simulink library "did"  (R2021b)
settings: Solver=VariableStepAuto  StartTime=0.0  StopTime=10.0  RelTol=1e-3
undefined symbols (not defined in the file): ADID_DODRange_pct, ADID_SOCRange_pct, ADID_TempRange_C, DiscIntNeverNeededParam, ENUM_CHRGPLUGSTA_AC, ENUM_CHRGPLUGSTA_DC, ENUM_CHRGPLUGSTA_NONE, ENUM_DRIVETRAIN_AWD, ENUM_DRIVETRAIN_FWD, ENUM_DRIVETRAIN_RWD, ENUM_EXTCHRGSTS_CHARGING, ENUM_OBCV2LSTA_WORKING, ENUM_PWRSTASW_READY, ENUM_VEHICLETYPE_D21, ENUM_VEHICLETYPE_D31F25, ENUM_VEHICLETYPE_D31HAWD, ENUM_VEHICLETYPE_D31HRWD, HOUR2SEC, HUNDRED, KDID_CPSAVehSpdThres_kph, KDID_DIDModelVersion_raw, KDID_DoDChrgCycle_s, KDID_FiveKmEquivEnergy_Wh, KDID_FlashInitDIDModelVersion_raw, KDID_IPSAVehSpdThres_kph, KDID_PropActiveTripThres_s, KDID_PSARResetThres_sec, KDID_RESSCNTSDODRNGAXIS_enum, KDID_RESSTIMESOCRNGAXIS_enum, KDID_RESSTTEMPRNGAXIS_enum, KDID_WarnUpPropActiveThres_s, KDID_WarnUpVehOperIdleThres_mph, KDID_WarnUpVehOperIdleThres_s, KDID_WarnUpVehOperThres_mph, KDID_WarnUpVehOperThres_s, KPH2MPH, KXX2XX, MINUSONE_FLOAT, ONE_FLOAT, ONE_INT, ONE_INT16, ONE_PERCENT, TRUE, UINT16_MAX, UINT32_MAX, XX2KXX, ZERO_FLOAT, ZERO_INT, ZERO_INT16, ZERO_INT32
libraries: hcu_lib x112, simulink x10, nmm x1
(part 3 of 4)

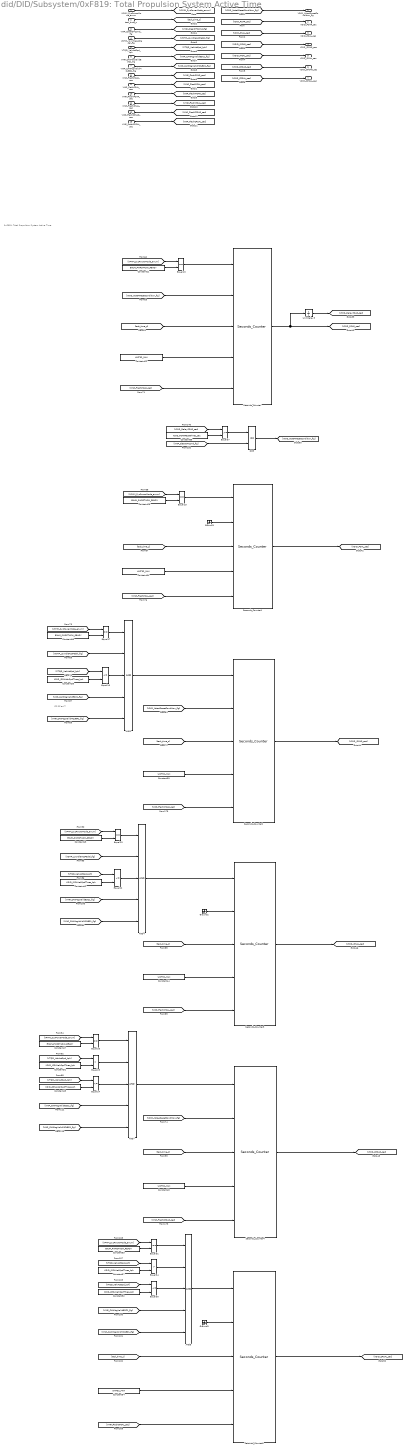
== system did/DID/Subsystem/0xF819: Total Propulsion System Active Time ==
  note: CS RC err??
  note: 0xF819: Total Propulsion System Active Time
  VPMM_SysPowerMode_enum : Inport
  task_time_s : Inport  Port=2
  VINP_ClearDTCcmd_flg : Inport  Port=3
  VDHP_LowIdleAccPedal_flg : Inport  Port=4
  VTQD_VehActSpd_kph : Inport  Port=5
  VINP_CANMsgValidESC1_flg : Inport  Port=6
  VINP_CANMsgValidMCUBR1_flg : Inport  Port=7
  VINP_FlashPSAR_sec : Inport  Port=8
  VINP_FlashPSAL_sec : Inport  Port=9
  VINP_FlashIPSAR_sec : Inport  Port=10
  VINP_FlashIPSAL_sec : Inport  Port=11
  VINP_FlashCPSAR_sec : Inport  Port=12
  VINP_FlashCPSAL_sec : Inport  Port=13
  AND{1,4..5,7} (4 alike) : Logic  Inputs=5  AllPortsSameDT=off  OutDataTypeStr=boolean
  Constant{21,26,36,43,47,53} (6 alike) : Constant  Value=ENUM_PWRSTASW_READY
  Constant{22,34,39,44,48,54} (6 alike) : Constant  Value=UINT32_MAX
  Constant{35,42,51,57} (4 alike) : Constant  Value=KDID_IPSAVehSpdThres_kph
  Constant45 : Constant  Value=KDID_CPSAVehSpdThres_kph
  Constant52 : Constant  Value=KDID_CPSAVehSpdThres_kph
  Constant65 : Constant  Value=KDID_PSARResetThres_sec
  Equal{13,15,17,23,26,31} (6 alike) : RelationalOperator  Operator===  OutDataTypeStr=boolean  RndMeth=Simplest
  Equal{16,22,24,30} (4 alike) : RelationalOperator  Operator=<=  OutDataTypeStr=boolean  RndMeth=Simplest
  Equal29 : RelationalOperator  Operator=>  OutDataTypeStr=boolean  RndMeth=Simplest
  Equal34 : RelationalOperator  Operator=>  OutDataTypeStr=boolean  RndMeth=Simplest
  Equal37 : RelationalOperator  OutDataTypeStr=boolean  RndMeth=Simplest
  Ground1 : Ground
  Ground2 : Ground
  Ground3 : Ground
  OR5 : Logic  Operator=OR  AllPortsSameDT=off  OutDataTypeStr=boolean
  Seconds_Counter{,1..5} (6 alike) : hcu_lib/Basic_Blocks/Seconds_Counter
  Unit Delay3 : UnitDelay  SampleTime=-1  HasFrameUpgradeWarning=on
  VDID_NoteAResetCondition_flg : Outport
  VDID_PSAR_sec : Outport  Port=2
  VDID_PSAL_sec : Outport  Port=3
  VDID_IPSAR_sec : Outport  Port=4
  VDID_IPSAL_sec : Outport  Port=5
  VDID_CPSAR_sec : Outport  Port=6
  VDID_CPSAL_sec : Outport  Port=7
  wires:
  Seconds_Counter3/1 -> [VDID_IPSAL_sec]
  [VDID_NoteAResetCondition_flg] -> Seconds_Counter4/2
  [VDID_NoteAResetCondition_flg] -> Seconds_Counter2/2
  Equal24/1 -> AND7/3
  [VINP_CANMsgValidMCUBR1_flg] -> AND7/5
  Constant42/1 -> Equal22/2
  Constant34/1 -> Seconds_Counter1/4
  [task_time_s] -> Seconds_Counter/3
  Equal16/1 -> AND1/3
  [task_time_s] -> Seconds_Counter2/3
  Equal17/1 -> AND1/1
  Ground2/1 -> Seconds_Counter3/2
  [VINP_ClearDTCcmd_flg] -> OR5/2
  AND1/1 -> Seconds_Counter2/1
  Equal31/1 -> AND5/1
  Constant51/1 -> Equal29/2
  [VINP_CANMsgValidMCUBR1_flg] -> AND1/5
  [VPMM_SysPowerMode_enum] -> Equal17/1
  [VDID_NoteAResetCondition_flg] -> Seconds_Counter/2
  [task_time_s] -> Seconds_Counter5/3
  Equal37/1 -> OR5/1
  [VINP_CANMsgValidESC1_flg] -> AND4/4
  [VDID_DelayPSAR_sec] -> Equal37/1
  Constant36/1 -> Equal17/2
  Constant47/1 -> Equal26/2
  [VTQD_VehActSpd_kph] -> Equal24/1
  Constant22/1 -> Seconds_Counter/4
  OR5/1 -> [VDID_NoteAResetCondition_flg]
  [VINP_FlashPSAL_sec] -> Seconds_Counter1/5
  Constant35/1 -> Equal16/2
  [VINP_FlashPSAR_sec] -> Seconds_Counter/5
  Constant54/1 -> Seconds_Counter5/4
  Seconds_Counter/1 -> Unit Delay3/1, [VDID_PSAR_sec]
  Equal15/1 -> Seconds_Counter1/1
  [VINP_CANMsgValidESC1_flg] -> AND5/4
  Equal22/1 -> AND4/3
  [VINP_CANMsgValidESC1_flg] -> AND7/4
  [VDHP_LowIdleAccPedal_flg] -> AND4/2
  [VINP_FlashCPSAR_sec] -> Seconds_Counter4/5
  Seconds_Counter5/1 -> [VDID_CPSAL_sec]
  [VINP_FlashIPSAL_sec] -> Seconds_Counter3/5
  Equal29/1 -> AND7/2
  [VPMM_SysPowerMode_enum] -> Equal31/1
  [VINP_FlashIPSAR_sec] -> Seconds_Counter2/5
  Constant65/1 -> Equal37/2
  [task_time_s] -> Seconds_Counter1/3
  Equal34/1 -> AND5/2
  Seconds_Counter1/1 -> [VDID_PSAL_sec]
  Constant57/1 -> Equal34/2
  [VTQD_VehActSpd_kph] -> Equal29/1
  AND5/1 -> Seconds_Counter5/1
  [VPMM_SysPowerMode_enum] -> Equal23/1
  Ground1/1 -> Seconds_Counter1/2
  [VINP_FlashCPSAL_sec] -> Seconds_Counter5/5
  Equal26/1 -> AND7/1
  [VTQD_VehActSpd_kph] -> Equal16/1
  [VINP_CANMsgValidMCUBR1_flg] -> AND5/5
  Unit Delay3/1 -> [VDID_DelayPSAR_sec]
  [task_time_s] -> Seconds_Counter4/3
  [VDHP_LowIdleAccPedal_flg] -> AND1/2
  [VPMM_SysPowerMode_enum] -> Equal13/1
  Constant52/1 -> Equal30/2
  Constant26/1 -> Equal15/2
  [VPMM_SysPowerMode_enum] -> Equal15/1
  Constant39/1 -> Seconds_Counter2/4
  [task_time_s] -> Seconds_Counter3/3
  Constant45/1 -> Equal24/2
  Seconds_Counter2/1 -> [VDID_IPSAR_sec]
  Constant44/1 -> Seconds_Counter3/4
  Equal13/1 -> Seconds_Counter/1
  Constant48/1 -> Seconds_Counter4/4
  [VINP_CANMsgValidESC1_flg] -> AND1/4
  [VINP_CANMsgValidMCUBR1_flg] -> AND4/5
  Ground3/1 -> Seconds_Counter5/2
  [VPMM_SysPowerMode_enum] -> Equal26/1
  [VTQD_VehActSpd_kph] -> Equal30/1
  [VTQD_VehActSpd_kph] -> Equal22/1
  AND4/1 -> Seconds_Counter3/1
  Equal23/1 -> AND4/1
  Constant53/1 -> Equal31/2
  Equal30/1 -> AND5/3
  [VTQD_VehActSpd_kph] -> Equal34/1
  Constant43/1 -> Equal23/2
  AND7/1 -> Seconds_Counter4/1
  Seconds_Counter4/1 -> [VDID_CPSAR_sec]
  Constant21/1 -> Equal13/2
  VPMM_SysPowerMode_enum/1 -> [VPMM_SysPowerMode_enum]
  task_time_s/1 -> [task_time_s]
  VINP_ClearDTCcmd_flg/1 -> [VINP_ClearDTCcmd_flg]
  VDHP_LowIdleAccPedal_flg/1 -> [VDHP_LowIdleAccPedal_flg]
  VINP_FlashPSAR_sec/1 -> [VINP_FlashPSAR_sec]
  VINP_CANMsgValidMCUBR1_flg/1 -> [VINP_CANMsgValidMCUBR1_flg]
  VINP_CANMsgValidESC1_flg/1 -> [VINP_CANMsgValidESC1_flg]
  VTQD_VehActSpd_kph/1 -> [VTQD_VehActSpd_kph]
  VINP_FlashIPSAR_sec/1 -> [VINP_FlashIPSAR_sec]
  VINP_FlashIPSAL_sec/1 -> [VINP_FlashIPSAL_sec]
  VINP_FlashCPSAR_sec/1 -> [VINP_FlashCPSAR_sec]
  VINP_FlashCPSAL_sec/1 -> [VINP_FlashCPSAL_sec]
  VINP_FlashPSAL_sec/1 -> [VINP_FlashPSAL_sec]
  [VDID_NoteAResetCondition_flg] -> VDID_NoteAResetCondition_flg/1
  [VDID_PSAR_sec] -> VDID_PSAR_sec/1
  [VDID_IPSAR_sec] -> VDID_IPSAR_sec/1
  [VDID_PSAL_sec] -> VDID_PSAL_sec/1
  [VDID_CPSAR_sec] -> VDID_CPSAR_sec/1
  [VDID_CPSAL_sec] -> VDID_CPSAL_sec/1
  [VDID_IPSAL_sec] -> VDID_IPSAL_sec/1

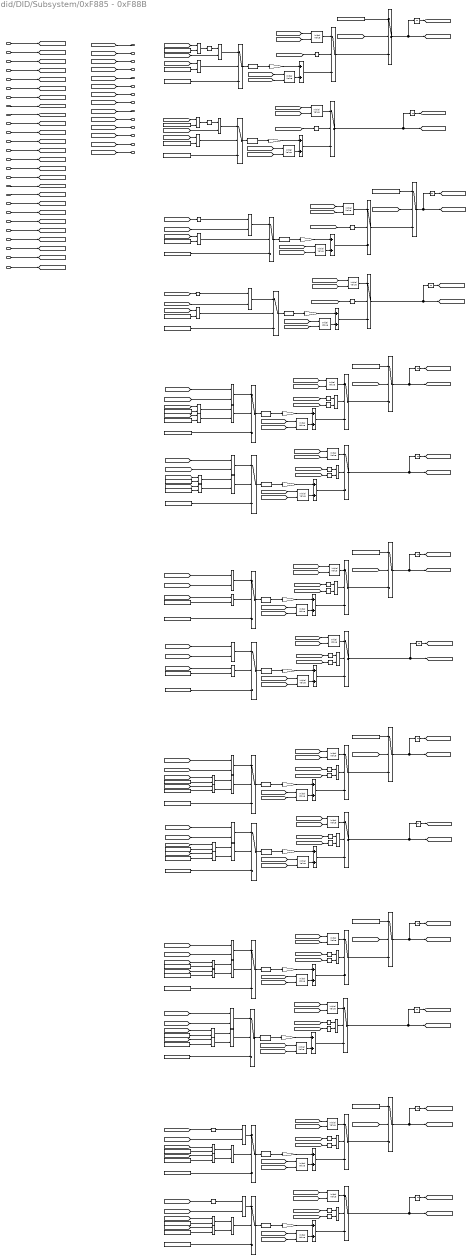
== system did/DID/Subsystem/0xF885 - 0xF88B ==
  note: 0xF88B: Total battery energy supplied to an off-board usage during propulsion system non-active operation
  note: 0xF88A: Total grid energy into the vehicle from off-board AC charging
  note: 0xF889: Total grid energy into the battery from off-board direct current (DC) charging
  note: 0xF887: Total energy into battery during propulsion system active
  note: 0xF888: Total grid energy into the battery during off-board charging
  note: 0xF886: Total net energy consumed in propulsion system active operation
  note: 0xF885: Total net battery current in propulsion system active operation
  VDID_HVBattCurr_A : Inport
  task_time_s : Inport  Port=2
  VPMM_SysPowerMode_enum : Inport  Port=3
  VINP_FlashTNBCPSAR_Ahr : Inport  Port=4
  VINP_CANMsgValidBMS1_flg : Inport  Port=5
  VDID_NoteAResetCondition_flg : Inport  Port=6
  VINP_FlashTNBCPSAL_Ahr : Inport  Port=7
  VDID_HVBattPwrDischrg_kW : Inport  Port=8
  VINP_FlashTNECPSAR_kWh : Inport  Port=9
  VINP_FlashTNECPSAL_kWh : Inport  Port=10
  VDID_HVBattPwrChrg_kW : Inport  Port=11
  VINP_ChrgPlugSta_enum : Inport  Port=12
  VINP_FlashTEBPSAR_kWh : Inport  Port=13
  VINP_CANMsgValidBMS6_flg : Inport  Port=14
  VINP_FlashTEBPSAL_kWh : Inport  Port=15
  VINP_ExtChrgSta_enum : Inport  Port=16
  VINP_FlashTGEOVCR_kWh : Inport  Port=17
  VINP_FlashTGEOVCL_kWh : Inport  Port=18
  VINP_FlashGECHGOVCDCR_kWh : Inport  Port=19
  VINP_FlashGECHGOVCDCL_kWh : Inport  Port=20
  VINP_FlashGECHGOVCACR_kWh : Inport  Port=21
  VINP_FlashGECHGOVCACL_kWh : Inport  Port=22
  VINP_FlashRESSV2XENNONPSAR_kWh : Inport  Port=23
  VINP_FlashRESSV2XENNONPSAL_kWh : Inport  Port=24
  VINP_CANMsgValidCCU2_flg : Inport  Port=25
  VINP_OBCV2LSta_enum : Inport  Port=26
  Abs{,1,4..7} (6 alike) : Abs
  Add{4..5,7..8,11..20} (14 alike) : Sum
  Constant{62,68..69,71..73,76..77,80..81,83,85,87..88,90,93,95,98,100,103,106,108,111} (23 alike) : Constant  Value=ZERO_FLOAT
  Constant{63,70,74..75,89,91,99,101} (8 alike) : Constant  Value=ENUM_PWRSTASW_READY
  Constant102 : Constant  Value=ENUM_OBCV2LSTA_WORKING
  Constant104 : Constant  Value=ENUM_OBCV2LSTA_WORKING
  Constant{78,82,84,86,107,109} (6 alike) : Constant  Value=ENUM_EXTCHRGSTS_CHARGING
  Constant110 : Constant  Value=ENUM_CHRGPLUGSTA_DC
  Constant41 : Constant  Value=ENUM_CHRGPLUGSTA_DC
  Constant92 : Constant  Value=ENUM_CHRGPLUGSTA_NONE
  Constant94 : Constant  Value=ENUM_CHRGPLUGSTA_NONE
  Constant96 : Constant  Value=ENUM_CHRGPLUGSTA_AC
  Constant97 : Constant  Value=ENUM_CHRGPLUGSTA_AC
  Data Type Conversion{12,15..22,24,26..28,30} (14 alike) : DataTypeConversion  OutDataTypeStr=single
  Equal{21,25,27..28,32..33,35..36,38..42,44..50} (20 alike) : RelationalOperator  Operator===  OutDataTypeStr=boolean  RndMeth=Simplest
  Equal43 : RelationalOperator  Operator=~=  OutDataTypeStr=boolean  RndMeth=Simplest
  Equal51 : RelationalOperator  Operator=~=  OutDataTypeStr=boolean  RndMeth=Simplest
  Gain{9..13,15..18,22..26} (14 alike) : Gain  Gain=1/HOUR2SEC
  Initial Value{1..28} (28 alike) : hcu_lib/Basic_Blocks/Initial Value
  Logical Operator{7..10,13,16..17,19,21,23} (10 alike) : Logic  Operator=OR  AllPortsSameDT=off  OutDataTypeStr=boolean
  Logical Operator{11..12,14..15,18,20,22,24} (8 alike) : Logic  AllPortsSameDT=off  OutDataTypeStr=boolean
  Min : MinMax  Inputs=2
  Min1 : MinMax  Inputs=2
  NOT{1,4..5,7..27} (24 alike) : Logic  Operator=NOT  AllPortsSameDT=off  OutDataTypeStr=boolean
  Product{5..13,16,19..20,23..24} (14 alike) : Product
  Switch{14..15,17..20,24..52} (35 alike) : Switch  Criteria=u2 > Threshold
  Unit Delay{7,9,15..19,21,24..25,28..31} (14 alike) : UnitDelay  SampleTime=-1  HasFrameUpgradeWarning=on
  VDID_TNBCPSAR_Ahr : Outport
  VDID_TNBCPSAL_Ahr : Outport  Port=2
  VDID_TNECPSAR_kWh : Outport  Port=3
  VDID_TNECPSAL_kWh : Outport  Port=4
  VDID_TEBPSAR_kWh : Outport  Port=5
  VDID_TEBPSAL_kWh : Outport  Port=6
  VDID_TGEOVCR_kWh : Outport  Port=7
  VDID_TGEOVCL_kWh : Outport  Port=8
  VDID_GECHGOVCDCR_kWh : Outport  Port=9
  VDID_GECHGOVCDCL_kWh : Outport  Port=10
  VDID_GECHGOVCACR_kWh : Outport  Port=11
  VDID_GECHGOVCACL_kWh : Outport  Port=12
  VDID_RESSV2XENNONPSAR_kWh : Outport  Port=13
  VDID_RESSV2XENNONPSAL_kWh : Outport  Port=14
  wires:
  Equal48/1 -> Logical Operator24/1
  Unit Delay24/1 -> [VINP_DelayGECHGOVCDCR_kWh]
  Add16/1 -> Switch45/3
  Gain9/1 -> Add4/1
  NOT24/1 -> Logical Operator17/2
  Constant102/1 -> Equal40/2
  Switch44/1 -> Data Type Conversion20/1
  [VINP_DelayRESSV2XENNONPSAL_kWh] -> Initial Value26/2
  Logical Operator17/1 -> Switch46/2
  Equal51/1 -> Logical Operator15/1
  [VINP_CANMsgValidBMS6_flg] -> NOT25/1
  [VPMM_SysPowerMode_enum] -> Equal33/1
  Switch46/1 -> [VDID_RESSV2XENNONPSAL_kWh], Unit Delay15/1
  Logical Operator14/1 -> Switch41/2
  [VINP_ChrgPlugSta_enum] -> Equal50/1
  Switch36/1 -> Data Type Conversion19/1
  Add4/1 -> Switch27/3
  Unit Delay18/1 -> [VINP_DelayTNECPSAL_kWh]
  Constant100/1 -> Switch43/3
  [VINP_CANMsgValidCCU2_flg] -> NOT21/1
  [VINP_OBCV2LSta_enum] -> Equal39/1
  Constant103/1 -> Switch41/3
  Initial Value26/1 -> Add20/2
  Initial Value20/1 -> Add11/2
  Initial Value23/1 -> Add19/2
  [VINP_CANMsgValidBMS1_flg] -> NOT24/1
  Constant86/1 -> Equal47/2
  Gain22/1 -> Add16/1
  Gain12/1 -> Add20/1
  Equal42/1 -> Switch17/2
  [VINP_DelayTNBCPSAL_Ahr] -> Initial Value9/2
  Logical Operator15/1 -> Switch43/2
  Constant83/1 -> Switch29/3
  Product12/1 -> Switch34/1
  [VINP_OBCV2LSta_enum] -> Equal40/1
  NOT21/1 -> Logical Operator17/1
  NOT1/1 -> Switch25/2
  Data Type Conversion30/1 -> Gain12/1
  Equal35/1 -> Logical Operator11/2
  Switch41/1 -> Data Type Conversion30/1
  Abs5/1 -> Product7/1
  Constant81/1 -> Switch28/1
  Constant63/1 -> Equal21/2
  NOT10/1 -> Logical Operator7/1
  Data Type Conversion20/1 -> Gain24/1
  [VINP_DelayRESSV2XENNONPSAR_kWh] -> Initial Value25/2
  Unit Delay15/1 -> [VINP_DelayRESSV2XENNONPSAL_kWh]
  [VINP_FlashRESSV2XENNONPSAL_kWh] -> Initial Value26/1
  [task_time_s] -> Product13/2
  Add20/1 -> Switch46/3
  [task_time_s] -> Product23/2
  [VINP_DelayTGEOVCL_kWh] -> Initial Value20/2
  Product20/1 -> Switch51/1
  NOT25/1 -> Logical Operator19/1
  Abs1/1 -> Product5/1
  [VINP_DelayGECHGOVCDCR_kWh] -> Initial Value21/2
  Switch33/1 -> Switch30/3
  Constant104/1 -> Equal39/2
  Switch45/1 -> Switch42/3
  Equal49/1 -> Logical Operator22/2
  Product23/1 -> Switch41/1
  [VINP_CANMsgValidBMS1_flg] -> NOT23/1
  [VPMM_SysPowerMode_enum] -> Equal51/1
  [VINP_CANMsgValidBMS6_flg] -> NOT10/1
  Equal39/1 -> Logical Operator14/2
  Constant99/1 -> Equal51/2
  [VPMM_SysPowerMode_enum] -> Equal43/1
  [task_time_s] -> Product24/2
  Constant101/1 -> Equal43/2
  Initial Value21/1 -> Add17/2
  [VDID_NoteAResetCondition_flg] -> Switch14/2
  Switch38/1 -> Unit Delay24/1, [VDID_GECHGOVCDCR_kWh]
  Equal43/1 -> Logical Operator14/1
  Initial Value13/1 -> Add7/2
  NOT12/1 -> Logical Operator9/2
  Min1/1 -> Abs1/1
  [task_time_s] -> Product20/2
  NOT22/1 -> Logical Operator16/1
  Constant68/1 -> Min/2
  Equal40/1 -> Logical Operator15/2
  Constant69/1 -> Min1/2
  Gain18/1 -> Add8/1
  Constant74/1 -> Equal41/2
  Data Type Conversion26/1 -> Gain22/1
  Data Type Conversion27/1 -> Gain18/1
  NOT23/1 -> Logical Operator16/2
  Constant98/1 -> Switch42/1
  [task_time_s] -> Product7/2
  NOT7/1 -> Switch27/2
  Switch31/1 -> Data Type Conversion17/1
  Switch43/1 -> Data Type Conversion26/1
  Initial Value22/1 -> Add15/2
  [VINP_DelayGECHGOVCDCL_kWh] -> Initial Value22/2
  Equal27/1 -> Switch29/2
  [task_time_s] -> Product6/2
  Constant92/1 -> Equal35/2
  [VINP_FlashTNECPSAL_kWh] -> Initial Value14/1
  NOT15/1 -> Logical Operator7/2
  [VINP_FlashRESSV2XENNONPSAR_kWh] -> Initial Value25/1
  Constant76/1 -> Switch17/3
  Data Type Conversion16/1 -> Gain23/1
  [VDID_HVBattPwrDischrg_kW] -> Abs5/1
  [VINP_CANMsgValidBMS1_flg] -> NOT12/1
  Initial Value19/1 -> Add12/2
  NOT26/1 -> Logical Operator19/2
  Switch42/1 -> Unit Delay9/1, [VDID_RESSV2XENNONPSAR_kWh]
  [VDID_NoteAResetCondition_flg] -> Switch48/2
  Add12/1 -> Switch35/3
  [VDID_HVBattCurr_A] -> Min/1
  [VDID_NoteAResetCondition_flg] -> Switch42/2
  [VINP_CANMsgValidCCU2_flg] -> NOT22/1
  Unit Delay9/1 -> [VINP_DelayRESSV2XENNONPSAR_kWh]
  Logical Operator16/1 -> Switch45/2
  Initial Value25/1 -> Add16/2
  Product16/1 -> Switch29/1
  Constant93/1 -> Switch34/3
  [VINP_ExtChrgSta_enum] -> Equal38/1
  [task_time_s] -> Product11/2
  Constant73/1 -> Switch26/3
  [VINP_CANMsgValidBMS1_flg] -> NOT4/1
  [VINP_CANMsgValidBMS6_flg] -> NOT27/1
  Switch40/1 -> Unit Delay25/1, [VDID_GECHGOVCACL_kWh]
  Add17/1 -> Switch47/3
  Constant41/1 -> Equal46/2
  Data Type Conversion28/1 -> Gain16/1
  [VPMM_SysPowerMode_enum] -> Equal42/1
  NOT16/1 -> Logical Operator21/2
  [VDID_HVBattPwrDischrg_kW] -> Abs7/1
  Abs7/1 -> Product23/1
  Switch27/1 -> [VDID_TNECPSAL_kWh], Unit Delay18/1
  Equal25/1 -> Switch24/2
  Abs6/1 -> Product24/1
  Abs/1 -> Product6/1
  [VDID_HVBattPwrDischrg_kW] -> Abs6/1
  Product24/1 -> Switch43/1
  Unit Delay19/1 -> [VINP_DelayTNBCPSAR_Ahr]
  Constant72/1 -> Switch15/1
  Switch26/1 -> Data Type Conversion15/1
  [VINP_DelayGECHGOVCACL_kWh] -> Initial Value24/2
  Switch18/1 -> Switch15/3
  Switch37/1 -> [VDID_TGEOVCL_kWh], Unit Delay30/1
  [VINP_DelayTNECPSAL_kWh] -> Initial Value14/2
  Add11/1 -> Switch37/3
  [VINP_ExtChrgSta_enum] -> Equal48/1
  Switch25/1 -> Switch14/3
  Equal33/1 -> Logical Operator11/1
  Switch52/1 -> Switch48/3
  Switch29/1 -> Data Type Conversion16/1
  Constant94/1 -> Equal36/2
  Data Type Conversion22/1 -> Gain26/1
  Data Type Conversion12/1 -> Gain10/1
  Switch28/1 -> [VDID_TGEOVCR_kWh], Unit Delay31/1
  Data Type Conversion18/1 -> Gain15/1
  Logical Operator11/1 -> Switch31/2
  [VDID_HVBattPwrChrg_kW] -> Product20/1
  [VINP_FlashTGEOVCR_kWh] -> Initial Value17/1
  Constant107/1 -> Equal38/2
  [VINP_ChrgPlugSta_enum] -> Equal36/1
  Constant71/1 -> Switch24/3
  Equal32/1 -> Logical Operator12/1
  [VDID_HVBattPwrDischrg_kW] -> Abs4/1
  Constant70/1 -> Equal25/2
  [VDID_NoteAResetCondition_flg] -> Switch15/2
  Equal36/1 -> Logical Operator12/2
  Logical Operator21/1 -> Switch50/2
  Equal41/1 -> Switch19/2
  Switch24/1 -> Data Type Conversion12/1
  Constant108/1 -> Switch44/3
  Initial Value10/1 -> Add8/2
  Gain10/1 -> Add7/1
  [VDID_HVBattCurr_A] -> Min1/1
  NOT4/1 -> Switch18/2
  [task_time_s] -> Product16/2
  [VINP_ExtChrgSta_enum] -> Equal27/1
  Constant80/1 -> Switch48/1
  NOT5/1 -> Switch20/2
  Min/1 -> Abs/1
  [VINP_DelayTNBCPSAR_Ahr] -> Initial Value10/2
  NOT13/1 -> Logical Operator10/1
  [VINP_FlashTNBCPSAR_Ahr] -> Initial Value10/1
  Switch30/1 -> [VDID_TEBPSAR_kWh], Unit Delay29/1
  Logical Operator9/1 -> Switch33/2
  Constant75/1 -> Equal42/2
  Switch35/1 -> [VDID_TEBPSAL_kWh], Unit Delay28/1
  Switch48/1 -> [VDID_GECHGOVCACR_kWh], Unit Delay7/1
  [task_time_s] -> Product8/2
  Data Type Conversion24/1 -> Gain25/1
  Switch19/1 -> Data Type Conversion28/1
  [VINP_CANMsgValidBMS1_flg] -> NOT16/1
  Logical Operator24/1 -> Switch39/2
  NOT8/1 -> Logical Operator8/1
  [VINP_CANMsgValidBMS1_flg] -> NOT7/1
  Data Type Conversion17/1 -> Gain17/1
  Add18/1 -> Switch40/3
  Abs4/1 -> Product8/1
  [VINP_CANMsgValidBMS1_flg] -> NOT5/1
  [VINP_ChrgPlugSta_enum] -> Equal46/1
  NOT17/1 -> Logical Operator13/1
  [VPMM_SysPowerMode_enum] -> Equal21/1
  [VPMM_SysPowerMode_enum] -> Equal32/1
  Initial Value14/1 -> Add4/2
  NOT9/1 -> Logical Operator8/2
  [VINP_DelayTEBPSAR_kWh] -> Initial Value18/2
  Equal28/1 -> Switch36/2
  Data Type Conversion15/1 -> Gain9/1
  Switch34/1 -> Data Type Conversion18/1
  [VINP_ExtChrgSta_enum] -> Equal28/1
  [task_time_s] -> Product5/2
  [VINP_ExtChrgSta_enum] -> Equal44/1
  Add14/1 -> Switch32/3
  Constant84/1 -> Equal28/2
  Constant111/1 -> Switch49/3
  Constant85/1 -> Switch36/3
  [VINP_DelayTEBPSAL_kWh] -> Initial Value19/2
  Initial Value17/1 -> Add14/2
  [VINP_FlashGECHGOVCDCR_kWh] -> Initial Value21/1
  Unit Delay31/1 -> [VINP_DelayTGEOVCR_kWh]
  [VINP_CANMsgValidBMS6_flg] -> NOT11/1
  Equal44/1 -> Logical Operator20/1
  Initial Value18/1 -> Add13/2
  [VINP_CANMsgValidBMS6_flg] -> NOT17/1
  Gain17/1 -> Add13/1
  [VINP_CANMsgValidBMS6_flg] -> NOT8/1
  Logical Operator8/1 -> Switch37/2
  Gain23/1 -> Add14/1
  Logical Operator19/1 -> Switch47/2
  [VDID_HVBattPwrChrg_kW] -> Product12/1
  NOT18/1 -> Logical Operator23/1
  Logical Operator10/1 -> Switch32/2
  [VDID_HVBattPwrChrg_kW] -> Product19/1
  Constant89/1 -> Equal33/2
  Logical Operator23/1 -> Switch52/2
  Unit Delay7/1 -> [VINP_DelayGECHGOVCACR_kWh]
  [VINP_FlashGECHGOVCACL_kWh] -> Initial Value24/1
  [VDID_NoteAResetCondition_flg] -> Switch28/2
  Logical Operator7/1 -> Switch35/2
  Gain13/1 -> Add11/1
  [VDID_HVBattPwrChrg_kW] -> Product16/1
  Equal47/1 -> Logical Operator22/1
  Constant87/1 -> Switch51/3
  [VINP_DelayGECHGOVCACR_kWh] -> Initial Value23/2
  [VINP_CANMsgValidBMS1_flg] -> NOT19/1
  Gain26/1 -> Add19/1
  Switch51/1 -> Data Type Conversion22/1
  [VINP_FlashGECHGOVCACR_kWh] -> Initial Value23/1
  [VINP_ExtChrgSta_enum] -> Equal47/1
  Add19/1 -> Switch52/3
  Constant96/1 -> Equal49/2
  Logical Operator22/1 -> Switch51/2
  [VINP_ChrgPlugSta_enum] -> Equal49/1
  Equal38/1 -> Logical Operator18/1
  Gain24/1 -> Add17/1
  NOT19/1 -> Logical Operator23/2
  Constant109/1 -> Equal44/2
  Unit Delay16/1 -> [VINP_DelayGECHGOVCDCL_kWh]
  Switch49/1 -> Data Type Conversion21/1
  [VDID_HVBattPwrChrg_kW] -> Product9/1
  Gain11/1 -> Add15/1
  Switch50/1 -> [VDID_GECHGOVCDCL_kWh], Unit Delay16/1
  NOT14/1 -> Logical Operator10/2
  [VINP_FlashGECHGOVCDCL_kWh] -> Initial Value22/1
  Gain16/1 -> Add5/1
  NOT27/1 -> Logical Operator21/1
  [task_time_s] -> Product9/2
  Data Type Conversion21/1 -> Gain11/1
  Add15/1 -> Switch50/3
  Unit Delay30/1 -> [VINP_DelayTGEOVCL_kWh]
  Logical Operator20/1 -> Switch49/2
  [VPMM_SysPowerMode_enum] -> Equal41/1
  Add8/1 -> Switch18/3
  Equal46/1 -> Logical Operator20/2
  Equal45/1 -> Logical Operator18/2
  Product13/1 -> Switch31/1
  Constant110/1 -> Equal45/2
  Constant77/1 -> Switch19/3
  Logical Operator18/1 -> Switch44/2
  [VINP_CANMsgValidBMS6_flg] -> NOT18/1
  Switch17/1 -> Data Type Conversion27/1
  Product8/1 -> Switch24/1
  [VINP_ChrgPlugSta_enum] -> Equal45/1
  Constant106/1 -> Switch38/1
  [task_time_s] -> Product10/2
  Switch14/1 -> Unit Delay21/1, [VDID_TNECPSAR_kWh]
  [VDID_HVBattPwrChrg_kW] -> Product10/1
  [VINP_FlashTNBCPSAL_Ahr] -> Initial Value9/1
  [VINP_CANMsgValidBMS1_flg] -> NOT9/1
  [VDID_NoteAResetCondition_flg] -> Switch38/2
  [VINP_CANMsgValidBMS1_flg] -> NOT26/1
  [VDID_HVBattPwrChrg_kW] -> Product13/1
  Switch47/1 -> Switch38/3
  Equal50/1 -> Logical Operator24/2
  Unit Delay25/1 -> [VINP_DelayGECHGOVCACL_kWh]
  Constant97/1 -> Equal50/2
  [task_time_s] -> Product19/2
  Initial Value24/1 -> Add18/2
  Logical Operator13/1 -> Switch40/2
  Switch39/1 -> Data Type Conversion24/1
  Gain25/1 -> Add18/1
  Gain15/1 -> Add12/1
  [VINP_CANMsgValidBMS1_flg] -> NOT20/1
  Constant95/1 -> Switch39/3
  Product19/1 -> Switch39/1
  Constant78/1 -> Equal48/2
  NOT20/1 -> Logical Operator13/2
  Unit Delay17/1 -> [VINP_DelayTNBCPSAL_Ahr]
  Initial Value9/1 -> Add5/2
  Switch15/1 -> [VDID_TNBCPSAR_Ahr], Unit Delay19/1
  Add5/1 -> Switch20/3
  Product5/1 -> Switch19/1
  Product6/1 -> Switch17/1
  Switch20/1 -> Unit Delay17/1, [VDID_TNBCPSAL_Ahr]
  [VINP_FlashTEBPSAL_kWh] -> Initial Value19/1
  [task_time_s] -> Product12/2
  [VINP_FlashTGEOVCL_kWh] -> Initial Value20/1
  [VINP_CANMsgValidBMS1_flg] -> NOT15/1
  Unit Delay28/1 -> [VINP_DelayTEBPSAL_kWh]
  Add13/1 -> Switch33/3
  [VINP_FlashTEBPSAR_kWh] -> Initial Value18/1
  Product9/1 -> Switch49/1
  Constant91/1 -> Equal32/2
  [VDID_NoteAResetCondition_flg] -> Switch30/2
  Constant88/1 -> Switch30/1
  Constant82/1 -> Equal27/2
  [VINP_CANMsgValidBMS1_flg] -> NOT14/1
  Equal21/1 -> Switch26/2
  Data Type Conversion19/1 -> Gain13/1
  Constant62/1 -> Switch14/1
  Logical Operator12/1 -> Switch34/2
  [VINP_DelayTNECPSAR_kWh] -> Initial Value13/2
  Unit Delay29/1 -> [VINP_DelayTEBPSAR_kWh]
  Add7/1 -> Switch25/3
  [VINP_FlashTNECPSAR_kWh] -> Initial Value13/1
  [VINP_CANMsgValidBMS1_flg] -> NOT1/1
  [VPMM_SysPowerMode_enum] -> Equal25/1
  Unit Delay21/1 -> [VINP_DelayTNECPSAR_kWh]
  Product7/1 -> Switch26/1
  [VINP_CANMsgValidBMS6_flg] -> NOT13/1
  Switch32/1 -> Switch28/3
  [VINP_ChrgPlugSta_enum] -> Equal35/1
  [VDID_HVBattPwrChrg_kW] -> Product11/1
  NOT11/1 -> Logical Operator9/1
  Constant90/1 -> Switch31/3
  [VINP_DelayTGEOVCR_kWh] -> Initial Value17/2
  Product10/1 -> Switch44/1
  Product11/1 -> Switch36/1
  VINP_FlashTNECPSAL_kWh/1 -> [VINP_FlashTNECPSAL_kWh]
  VINP_FlashTEBPSAR_kWh/1 -> [VINP_FlashTEBPSAR_kWh]
  VINP_CANMsgValidBMS6_flg/1 -> [VINP_CANMsgValidBMS6_flg]
  VINP_FlashTEBPSAL_kWh/1 -> [VINP_FlashTEBPSAL_kWh]
  VDID_HVBattPwrChrg_kW/1 -> [VDID_HVBattPwrChrg_kW]
  VINP_ChrgPlugSta_enum/1 -> [VINP_ChrgPlugSta_enum]
  VDID_HVBattPwrDischrg_kW/1 -> [VDID_HVBattPwrDischrg_kW]
  VPMM_SysPowerMode_enum/1 -> [VPMM_SysPowerMode_enum]
  VINP_FlashTNBCPSAL_Ahr/1 -> [VINP_FlashTNBCPSAL_Ahr]
  [VDID_TEBPSAR_kWh] -> VDID_TEBPSAR_kWh/1
  task_time_s/1 -> [task_time_s]
  [VDID_GECHGOVCDCR_kWh] -> VDID_GECHGOVCDCR_kWh/1
  [VDID_RESSV2XENNONPSAR_kWh] -> VDID_RESSV2XENNONPSAR_kWh/1
  VDID_HVBattCurr_A/1 -> [VDID_HVBattCurr_A]
  [VDID_GECHGOVCACR_kWh] -> VDID_GECHGOVCACR_kWh/1
  VDID_NoteAResetCondition_flg/1 -> [VDID_NoteAResetCondition_flg]
  [VDID_TNBCPSAR_Ahr] -> VDID_TNBCPSAR_Ahr/1
  [VDID_GECHGOVCDCL_kWh] -> VDID_GECHGOVCDCL_kWh/1
  [VDID_TGEOVCL_kWh] -> VDID_TGEOVCL_kWh/1
  [VDID_TNECPSAR_kWh] -> VDID_TNECPSAR_kWh/1
  [VDID_TGEOVCR_kWh] -> VDID_TGEOVCR_kWh/1
  [VDID_GECHGOVCACL_kWh] -> VDID_GECHGOVCACL_kWh/1
  VINP_FlashRESSV2XENNONPSAL_kWh/1 -> [VINP_FlashRESSV2XENNONPSAL_kWh]
  VINP_FlashRESSV2XENNONPSAR_kWh/1 -> [VINP_FlashRESSV2XENNONPSAR_kWh]
  VINP_CANMsgValidCCU2_flg/1 -> [VINP_CANMsgValidCCU2_flg]
  VINP_CANMsgValidBMS1_flg/1 -> [VINP_CANMsgValidBMS1_flg]
  VINP_FlashGECHGOVCACL_kWh/1 -> [VINP_FlashGECHGOVCACL_kWh]
  VINP_FlashTGEOVCR_kWh/1 -> [VINP_FlashTGEOVCR_kWh]
  [VDID_RESSV2XENNONPSAL_kWh] -> VDID_RESSV2XENNONPSAL_kWh/1
  VINP_FlashTNBCPSAR_Ahr/1 -> [VINP_FlashTNBCPSAR_Ahr]
  VINP_FlashGECHGOVCDCR_kWh/1 -> [VINP_FlashGECHGOVCDCR_kWh]
  [VDID_TEBPSAL_kWh] -> VDID_TEBPSAL_kWh/1
  VINP_FlashTGEOVCL_kWh/1 -> [VINP_FlashTGEOVCL_kWh]
  VINP_FlashGECHGOVCDCL_kWh/1 -> [VINP_FlashGECHGOVCDCL_kWh]
  VINP_ExtChrgSta_enum/1 -> [VINP_ExtChrgSta_enum]
  [VDID_TNBCPSAL_Ahr] -> VDID_TNBCPSAL_Ahr/1
  [VDID_TNECPSAL_kWh] -> VDID_TNECPSAL_kWh/1
  VINP_FlashGECHGOVCACR_kWh/1 -> [VINP_FlashGECHGOVCACR_kWh]
  VINP_FlashTNECPSAR_kWh/1 -> [VINP_FlashTNECPSAR_kWh]
  VINP_OBCV2LSta_enum/1 -> [VINP_OBCV2LSta_enum]
  [VINP_DelayTNBCPSAR_Ahr] -> Initial Value1/2
  [VINP_FlashTNBCPSAR_Ahr] -> Initial Value1/1
  Initial Value1/1 -> Switch18/1
  [VINP_DelayTNBCPSAL_Ahr] -> Initial Value2/2
  [VINP_FlashTNBCPSAL_Ahr] -> Initial Value2/1
  Initial Value2/1 -> Switch20/1
  [VINP_FlashTNECPSAR_kWh] -> Initial Value3/1
  [VINP_DelayTNECPSAR_kWh] -> Initial Value3/2
  Initial Value3/1 -> Switch25/1
  [VINP_DelayTNECPSAL_kWh] -> Initial Value4/2
  [VINP_FlashTNECPSAL_kWh] -> Initial Value4/1
  Initial Value4/1 -> Switch27/1
  [VINP_DelayTEBPSAR_kWh] -> Initial Value5/2
  [VINP_FlashTEBPSAR_kWh] -> Initial Value5/1
  Initial Value5/1 -> Switch33/1
  [VINP_FlashTEBPSAL_kWh] -> Initial Value6/1
  [VINP_DelayTEBPSAL_kWh] -> Initial Value6/2
  Initial Value6/1 -> Switch35/1
  [VINP_DelayTGEOVCR_kWh] -> Initial Value7/2
  [VINP_FlashTGEOVCR_kWh] -> Initial Value7/1
  Initial Value7/1 -> Switch32/1
  [VINP_DelayTGEOVCL_kWh] -> Initial Value8/2
  [VINP_FlashTGEOVCL_kWh] -> Initial Value8/1
  Initial Value8/1 -> Switch37/1
  [VINP_DelayGECHGOVCDCR_kWh] -> Initial Value11/2
  [VINP_FlashGECHGOVCDCR_kWh] -> Initial Value11/1
  Initial Value11/1 -> Switch47/1
  [VINP_DelayGECHGOVCDCL_kWh] -> Initial Value12/2
  [VINP_FlashGECHGOVCDCL_kWh] -> Initial Value12/1
  Initial Value12/1 -> Switch50/1
  [VINP_DelayGECHGOVCACR_kWh] -> Initial Value15/2
  [VINP_FlashGECHGOVCACR_kWh] -> Initial Value15/1
  Initial Value15/1 -> Switch52/1
  [VINP_DelayGECHGOVCACL_kWh] -> Initial Value16/2
  [VINP_FlashGECHGOVCACL_kWh] -> Initial Value16/1
  Initial Value16/1 -> Switch40/1
  [VINP_FlashRESSV2XENNONPSAR_kWh] -> Initial Value27/1
  [VINP_DelayRESSV2XENNONPSAR_kWh] -> Initial Value27/2
  Initial Value27/1 -> Switch45/1
  [VINP_FlashRESSV2XENNONPSAL_kWh] -> Initial Value28/1
  [VINP_DelayRESSV2XENNONPSAL_kWh] -> Initial Value28/2
  Initial Value28/1 -> Switch46/1

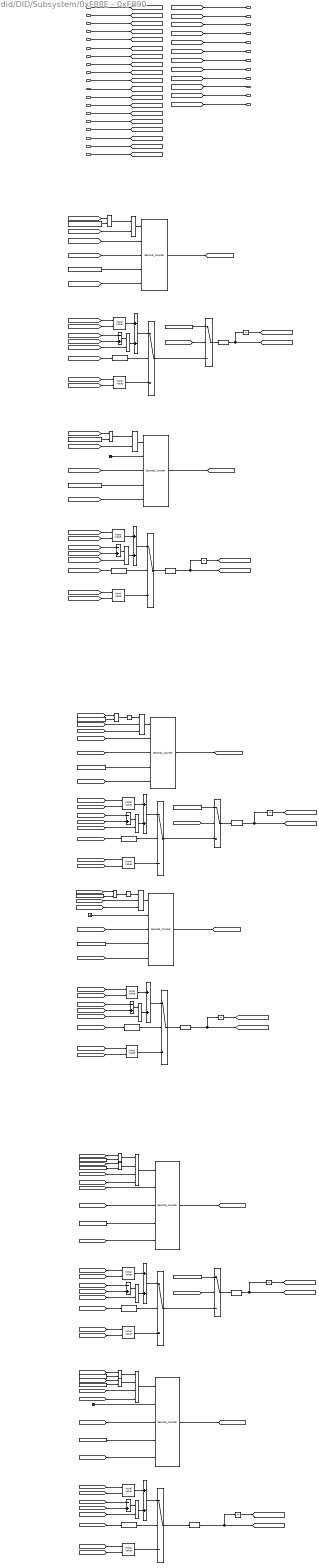
== system did/DID/Subsystem/0xF88E - 0xF890 ==
  note: 0xF88E: Average Battery Temperature during Propulsion System Active
  note: 0xF88F: Average Battery Temperature during Charging
  note: 0xF890: Average battery temperature while vehicle Off
  VPMM_SysPowerMode_enum : Inport
  VINP_CANMsgValidBMS4_flg : Inport  Port=2
  VINP_CANMsgValidBMS6_flg : Inport  Port=3
  VDID_NoteAResetCondition_flg : Inport  Port=4
  VINP_ChrgPlugSta_enum : Inport  Port=5
  task_time_s : Inport  Port=6
  VINP_CellTempAvg_C : Inport  Port=7
  VINP_FlashTempPSAR_sec : Inport  Port=8
  VDID_FlashAvgBattTempPSAR_C : Inport  Port=9
  VINP_FlashTempPSAL_sec : Inport  Port=10
  VDID_FlashAvgBattTempPSAL_C : Inport  Port=11
  VINP_FlashOVCR_sec : Inport  Port=12
  VDID_FlashAvgBattTempOVCR_C : Inport  Port=13
  VINP_FlashOVCL_sec : Inport  Port=14
  VDID_FlashAvgBattTempOVCL_C : Inport  Port=15
  VINP_FlashOFFR_sec : Inport  Port=16
  VDID_FlashAvgBattTempOFFR_C : Inport  Port=17
  VINP_FlashOFFL_sec : Inport  Port=18
  VDID_FlashAvgBattTempOFFL_C : Inport  Port=19
  AND11 : Logic  Inputs=3  AllPortsSameDT=off  OutDataTypeStr=boolean
  AND12 : Logic  Inputs=3  AllPortsSameDT=off  OutDataTypeStr=boolean
  AND13 : Logic  Inputs=4  AllPortsSameDT=off  OutDataTypeStr=boolean
  AND14 : Logic  Inputs=4  AllPortsSameDT=off  OutDataTypeStr=boolean
  AND3 : Logic  AllPortsSameDT=off  OutDataTypeStr=boolean
  AND9 : Logic  AllPortsSameDT=off  OutDataTypeStr=boolean
  Constant112 : Constant  Value=ZERO_FLOAT  OutDataTypeStr=single
  Constant{64,114,117,119,123,125} (6 alike) : Constant  Value=UINT32_MAX
  Constant{58,61,115..116} (4 alike) : Constant  Value=ENUM_CHRGPLUGSTA_NONE
  Constant118 : Constant  Value=ZERO_FLOAT  OutDataTypeStr=single
  Constant{120..122,124} (4 alike) : Constant  Value=ENUM_PWRSTASW_READY
  Constant55 : Constant  Value=ZERO_FLOAT  OutDataTypeStr=single
  Data Type Conversion{,1..5} (6 alike) : DataTypeConversion  OutDataTypeStr=single
  Divide{3..8} (6 alike) : Product  Inputs=*/
  Equal{52..55,58..59} (6 alike) : RelationalOperator  Operator===  OutDataTypeStr=boolean  RndMeth=Simplest
  Equal56 : RelationalOperator  Operator=~=  OutDataTypeStr=boolean  RndMeth=Simplest
  Equal57 : RelationalOperator  Operator=~=  OutDataTypeStr=boolean  RndMeth=Simplest
  Ground : Ground
  Ground4 : Ground
  Ground5 : Ground
  Initial Value{4..6,15..16,27..33} (12 alike) : hcu_lib/Basic_Blocks/Initial Value
  NOT28 : Logic  Operator=NOT  AllPortsSameDT=off  OutDataTypeStr=boolean
  NOT29 : Logic  Operator=NOT  AllPortsSameDT=off  OutDataTypeStr=boolean
  Real_DetectChange{,1..5} (6 alike) : hcu_lib/Basic_Blocks/Real_DetectChange
  Seconds_Counter{6..11} (6 alike) : hcu_lib/Basic_Blocks/Seconds_Counter
  Subtract{5,8,10..11,13..14} (6 alike) : Sum  Inputs=-+
  Subtract{4,7,9,12,15..16} (6 alike) : Sum
  Switch{5,23,53..59} (9 alike) : Switch  Criteria=u2 ~= 0
      settings: AttributesFormatString=<%<Criteria>>
  Unit Delay{10,12,22,26..27,32} (6 alike) : UnitDelay  SampleTime=-1  HasFrameUpgradeWarning=on
  VDID_AvgBattTempPSAR_C : Outport
  VDID_AvgBattTempPSAL_C : Outport  Port=2
  VDID_AvgBattTempOVCR_C : Outport  Port=3
  VDID_AvgBattTempOVCL_C : Outport  Port=4
  VDID_AvgBattTempOFFR_C : Outport  Port=5
  VDID_AvgBattTempOFFL_C : Outport  Port=6
  VDID_BattTempPSAR_sec : Outport  Port=7
  VDID_BattTempPSAL_sec : Outport  Port=8
  VDID_OVCR_sec : Outport  Port=9
  VDID_OVCL_sec : Outport  Port=10
  VDID_OFFR_sec : Outport  Port=11
  VDID_OFFL_sec : Outport  Port=12
  wires:
  Ground/1 -> Seconds_Counter7/2
  [task_time_s] -> Seconds_Counter11/3
  AND11/1 -> Seconds_Counter6/1
  Unit Delay26/1 -> [VDID_DelayAvgBattTempPSAR_C]
  [VDID_OFFL_sec] -> Real_DetectChange/1
  AND14/1 -> Seconds_Counter9/1
  [VDID_DelayAvgBattTempPSAL_C] -> Subtract8/1
  [VDID_DelayAvgBattTempOFFR_C] -> Initial Value30/2
  Subtract12/1 -> Switch57/1
  Divide5/1 -> Subtract9/2
  Switch58/1 -> Switch53/3
  [VINP_CellTempAvg_C] -> Subtract11/2
  [VDID_NoteAResetCondition_flg] -> Switch55/2
  [VDID_DelayAvgBattTempOVCR_C] -> Initial Value27/2
  Subtract9/1 -> Switch56/1
  Constant116/1 -> Equal54/2
  Initial Value5/1 -> Subtract4/1
  Constant114/1 -> Seconds_Counter7/4
  Subtract13/1 -> Divide7/1
  [VPMM_SysPowerMode_enum] -> Equal58/1
  Unit Delay27/1 -> [VDID_DelayAvgBattTempPSAL_C]
  [VDID_DelayAvgBattTempOVCL_C] -> Initial Value29/2
  Subtract16/1 -> Switch58/1
  Switch59/1 -> Data Type Conversion5/1
  Initial Value4/1 -> Switch23/3
  Initial Value15/1 -> Switch56/3
  Constant120/1 -> Equal56/2
  [VINP_FlashTempPSAL_sec] -> Seconds_Counter11/5
  Seconds_Counter10/1 -> [VDID_BattTempPSAR_sec]
  [task_time_s] -> Seconds_Counter8/3
  Initial Value16/1 -> Switch54/3
  Subtract7/1 -> Switch54/1
  [VDID_FlashAvgBattTempOVCR_C] -> Initial Value27/1
  [VDID_FlashAvgBattTempOFFR_C] -> Initial Value31/1
  Equal54/1 -> AND13/2
  Unit Delay22/1 -> [VDID_DelayAvgBattTempOFFR_C]
  [VDID_BattTempPSAR_sec] -> Real_DetectChange5/1
  Constant61/1 -> Equal52/2
  [VINP_CANMsgValidBMS4_flg] -> AND9/2
  Switch57/1 -> Data Type Conversion3/1
  [VDID_DelayAvgBattTempPSAR_C] -> Subtract5/1
  [VDID_OFFL_sec] -> Divide8/2
  Initial Value27/1 -> Subtract9/1
  Unit Delay32/1 -> [VDID_DelayAvgBattTempOVCR_C]
  [task_time_s] -> Seconds_Counter6/3
  Initial Value29/1 -> Subtract12/1
  [VINP_FlashOVCL_sec] -> Seconds_Counter7/5
  [VDID_FlashAvgBattTempOVCL_C] -> Initial Value29/1
  Unit Delay10/1 -> [VDID_DelayAvgBattTempOVCL_C]
  Seconds_Counter7/1 -> [VDID_OVCL_sec]
  Equal59/1 -> AND3/1
  [VDID_FlashAvgBattTempOFFL_C] -> Initial Value32/1
  Subtract10/1 -> Divide5/1
  [task_time_s] -> Seconds_Counter7/3
  Constant118/1 -> Switch53/1
  [VPMM_SysPowerMode_enum] -> Equal56/1
  Switch23/1 -> Switch5/3
  Divide7/1 -> Subtract16/2
  [VINP_ChrgPlugSta_enum] -> Equal54/1
  [VDID_DelayAvgBattTempOVCL_C] -> Initial Value28/2
  Divide3/1 -> Subtract4/2
  [VDID_OVCL_sec] -> Divide6/2
  [task_time_s] -> Seconds_Counter9/3
  Real_DetectChange2/1 -> Switch57/2
  AND12/1 -> Seconds_Counter7/1
  Subtract5/1 -> Divide3/1
  Subtract8/1 -> Divide4/1
  [VDID_DelayAvgBattTempOFFL_C] -> Initial Value32/2
  [VDID_DelayAvgBattTempOVCR_C] -> Initial Value15/2
  Divide4/1 -> Subtract7/2
  [VINP_CANMsgValidBMS4_flg] -> AND11/2
  [VDID_NoteAResetCondition_flg] -> Seconds_Counter8/2
  AND3/1 -> Seconds_Counter11/1
  [VDID_FlashAvgBattTempPSAL_C] -> Initial Value16/1
  [VINP_FlashOVCR_sec] -> Seconds_Counter6/5
  Switch55/1 -> Data Type Conversion2/1
  [VDID_DelayAvgBattTempPSAR_C] -> Initial Value5/2
  Switch56/1 -> Switch55/3
  [VDID_DelayAvgBattTempPSAL_C] -> Initial Value6/2
  Subtract4/1 -> Switch23/1
  [VINP_CellTempAvg_C] -> Subtract5/2
  Initial Value28/1 -> Switch57/3
  Equal52/1 -> NOT28/1
  Initial Value6/1 -> Subtract7/1
  [VDID_OVCR_sec] -> Real_DetectChange3/1
  Real_DetectChange5/1 -> Switch23/2
  [VDID_OFFR_sec] -> Real_DetectChange1/1
  [VDID_DelayAvgBattTempOFFR_C] -> Subtract13/1
  NOT29/1 -> AND12/1
  Constant55/1 -> Switch5/1
  [VINP_FlashOFFR_sec] -> Seconds_Counter8/5
  Seconds_Counter11/1 -> [VDID_BattTempPSAL_sec]
  Switch54/1 -> Data Type Conversion1/1
  [VINP_CellTempAvg_C] -> Subtract10/2
  [VDID_OVCR_sec] -> Divide5/2
  Constant123/1 -> Seconds_Counter10/4
  [VINP_CANMsgValidBMS4_flg] -> AND12/2
  [VINP_CellTempAvg_C] -> Subtract13/2
  [VINP_CANMsgValidBMS6_flg] -> AND14/4
  Constant58/1 -> Equal53/2
  NOT28/1 -> AND11/1
  [VDID_NoteAResetCondition_flg] -> Seconds_Counter10/2
  Constant112/1 -> Switch55/1
  [VDID_NoteAResetCondition_flg] -> Switch5/2
  Equal57/1 -> AND14/1
  Initial Value31/1 -> Subtract16/1
  Divide6/1 -> Subtract12/2
  Equal58/1 -> AND9/1
  [VINP_FlashOFFL_sec] -> Seconds_Counter9/5
  [VDID_FlashAvgBattTempOFFR_C] -> Initial Value30/1
  [VDID_FlashAvgBattTempPSAR_C] -> Initial Value4/1
  [VINP_CANMsgValidBMS6_flg] -> AND12/3
  Initial Value30/1 -> Switch58/3
  [VPMM_SysPowerMode_enum] -> Equal59/1
  [VDID_DelayAvgBattTempOVCL_C] -> Subtract11/1
  Unit Delay12/1 -> [VDID_DelayAvgBattTempOFFL_C]
  Ground5/1 -> Seconds_Counter9/2
  Constant119/1 -> Seconds_Counter9/4
  [VINP_ChrgPlugSta_enum] -> Equal55/1
  [VPMM_SysPowerMode_enum] -> Equal57/1
  Subtract11/1 -> Divide6/1
  [task_time_s] -> Seconds_Counter10/3
  Constant117/1 -> Seconds_Counter8/4
  [VDID_DelayAvgBattTempPSAL_C] -> Initial Value16/2
  [VDID_DelayAvgBattTempPSAR_C] -> Initial Value4/2
  [VDID_DelayAvgBattTempOFFL_C] -> Subtract14/1
  [VINP_CellTempAvg_C] -> Subtract14/2
  Divide8/1 -> Subtract15/2
  [VINP_CANMsgValidBMS4_flg] -> AND14/3
  [VINP_CANMsgValidBMS6_flg] -> AND11/3
  Seconds_Counter8/1 -> [VDID_OFFR_sec]
  Equal55/1 -> AND14/2
  [VINP_FlashTempPSAR_sec] -> Seconds_Counter10/5
  Equal53/1 -> NOT29/1
  [VDID_NoteAResetCondition_flg] -> Seconds_Counter6/2
  Switch53/1 -> Data Type Conversion4/1
  [VDID_FlashAvgBattTempPSAL_C] -> Initial Value6/1
  [VDID_DelayAvgBattTempOVCR_C] -> Subtract10/1
  [VINP_ChrgPlugSta_enum] -> Equal53/1
  [VDID_BattTempPSAR_sec] -> Divide3/2
  Constant115/1 -> Equal55/2
  [VDID_FlashAvgBattTempOVCL_C] -> Initial Value28/1
  Constant64/1 -> Seconds_Counter6/4
  Seconds_Counter9/1 -> [VDID_OFFL_sec]
  Constant124/1 -> Equal59/2
  Ground4/1 -> Seconds_Counter11/2
  AND9/1 -> Seconds_Counter10/1
  Seconds_Counter6/1 -> [VDID_OVCR_sec]
  Real_DetectChange/1 -> Switch59/2
  Equal56/1 -> AND13/1
  Real_DetectChange3/1 -> Switch56/2
  [VDID_BattTempPSAL_sec] -> Real_DetectChange4/1
  Real_DetectChange1/1 -> Switch58/2
  Real_DetectChange4/1 -> Switch54/2
  Initial Value33/1 -> Subtract15/1
  [VINP_CellTempAvg_C] -> Subtract8/2
  Constant125/1 -> Seconds_Counter11/4
  Constant122/1 -> Equal57/2
  [VINP_ChrgPlugSta_enum] -> Equal52/1
  [VDID_OFFR_sec] -> Divide7/2
  Constant121/1 -> Equal58/2
  [VDID_OVCL_sec] -> Real_DetectChange2/1
  [VDID_DelayAvgBattTempOFFR_C] -> Initial Value31/2
  [VINP_CANMsgValidBMS4_flg] -> AND3/2
  [VDID_FlashAvgBattTempOVCR_C] -> Initial Value15/1
  [VDID_FlashAvgBattTempPSAR_C] -> Initial Value5/1
  [VINP_CANMsgValidBMS4_flg] -> AND13/3
  AND13/1 -> Seconds_Counter8/1
  Initial Value32/1 -> Switch59/3
  [VDID_NoteAResetCondition_flg] -> Switch53/2
  Subtract14/1 -> Divide8/1
  [VINP_CANMsgValidBMS6_flg] -> AND13/4
  [VDID_DelayAvgBattTempOFFL_C] -> Initial Value33/2
  [VDID_BattTempPSAL_sec] -> Divide4/2
  [VDID_FlashAvgBattTempOFFL_C] -> Initial Value33/1
  Subtract15/1 -> Switch59/1
  VPMM_SysPowerMode_enum/1 -> [VPMM_SysPowerMode_enum]
  VINP_CANMsgValidBMS4_flg/1 -> [VINP_CANMsgValidBMS4_flg]
  VINP_CANMsgValidBMS6_flg/1 -> [VINP_CANMsgValidBMS6_flg]
  VDID_NoteAResetCondition_flg/1 -> [VDID_NoteAResetCondition_flg]
  VINP_ChrgPlugSta_enum/1 -> [VINP_ChrgPlugSta_enum]
  task_time_s/1 -> [task_time_s]
  VINP_CellTempAvg_C/1 -> [VINP_CellTempAvg_C]
  VINP_FlashTempPSAR_sec/1 -> [VINP_FlashTempPSAR_sec]
  VDID_FlashAvgBattTempPSAR_C/1 -> [VDID_FlashAvgBattTempPSAR_C]
  VINP_FlashTempPSAL_sec/1 -> [VINP_FlashTempPSAL_sec]
  VDID_FlashAvgBattTempPSAL_C/1 -> [VDID_FlashAvgBattTempPSAL_C]
  VINP_FlashOVCR_sec/1 -> [VINP_FlashOVCR_sec]
  VDID_FlashAvgBattTempOVCR_C/1 -> [VDID_FlashAvgBattTempOVCR_C]
  VINP_FlashOVCL_sec/1 -> [VINP_FlashOVCL_sec]
  VDID_FlashAvgBattTempOVCL_C/1 -> [VDID_FlashAvgBattTempOVCL_C]
  VINP_FlashOFFR_sec/1 -> [VINP_FlashOFFR_sec]
  VDID_FlashAvgBattTempOFFR_C/1 -> [VDID_FlashAvgBattTempOFFR_C]
  VINP_FlashOFFL_sec/1 -> [VINP_FlashOFFL_sec]
  VDID_FlashAvgBattTempOFFL_C/1 -> [VDID_FlashAvgBattTempOFFL_C]
  [VDID_AvgBattTempPSAR_C] -> VDID_AvgBattTempPSAR_C/1
  [VDID_AvgBattTempOFFL_C] -> VDID_AvgBattTempOFFL_C/1
  [VDID_AvgBattTempOFFR_C] -> VDID_AvgBattTempOFFR_C/1
  [VDID_AvgBattTempOVCL_C] -> VDID_AvgBattTempOVCL_C/1
  [VDID_AvgBattTempOVCR_C] -> VDID_AvgBattTempOVCR_C/1
  [VDID_AvgBattTempPSAL_C] -> VDID_AvgBattTempPSAL_C/1
  Switch5/1 -> Data Type Conversion/1
  Data Type Conversion/1 -> Unit Delay26/1, [VDID_AvgBattTempPSAR_C]
  Data Type Conversion1/1 -> [VDID_AvgBattTempPSAL_C], Unit Delay27/1
  Data Type Conversion2/1 -> [VDID_AvgBattTempOVCR_C], Unit Delay32/1
  Data Type Conversion3/1 -> [VDID_AvgBattTempOVCL_C], Unit Delay10/1
  Data Type Conversion4/1 -> [VDID_AvgBattTempOFFR_C], Unit Delay22/1
  Data Type Conversion5/1 -> [VDID_AvgBattTempOFFL_C], Unit Delay12/1
  [VDID_BattTempPSAR_sec] -> VDID_BattTempPSAR_sec/1
  [VDID_OVCR_sec] -> VDID_OVCR_sec/1
  [VDID_BattTempPSAL_sec] -> VDID_BattTempPSAL_sec/1
  [VDID_OVCL_sec] -> VDID_OVCL_sec/1
  [VDID_OFFR_sec] -> VDID_OFFR_sec/1
  [VDID_OFFL_sec] -> VDID_OFFL_sec/1
